simulink model "sim_sil_target_block"  (Simulink 8.1)
settings: Solver=FixedStepDiscrete  StartTime=0.0  StopTime=10.0  FixedStep=Auto  RelTol=1e-3  SampleTimeConstraint=STIndependent
undefined symbols (not defined in the file or in its folder): A10, A13, A14, B, B13, C6, D, D11, D4, K4, L3, PA10, PA11, PA12, PA13, PC6, PC7, R10
libraries: rappid_564xl_ec_toolbox x4, BAMLIB564xL x1
settings Model: Creator=evarshavskaya  LastModifiedBy=evarshavskaya  SimulationMode=software-in-the-loop (sil)
settings DataIOCC: ExternalInput=off  InitialState=off  SaveOutput=off  SignalLogging=off  SaveTime=off
settings OptimizationCC: InlineParams=on  OptimizeModelRefInitCode=on  LifeSpan=1
settings DebuggingCC: InheritedTsInSrcMsg=none  SingleTaskRateTransMsg=error  UnconnectedInputMsg=error  UnconnectedOutputMsg=error  UnconnectedLineMsg=error  UnknownTsInhSupMsg=error
settings HardwareCC: ProdIntDivRoundTo=Zero  ProdEndianess=LittleEndian  ProdHWDeviceType=Generic->Custom
settings ModelReferenceCC: ModelReferenceNumInstancesAllowed=Single
settings RTWCC: SystemTargetFile=ert.tlc  TemplateMakefile=ert_default_tmf  PostCodeGenCommand=rappid_analyzegencode(buildInfo)  Description=Embedded Coder  ProcessScript=ert_make_rtw_hook  PortableWordSizes=on  GenerateErtSFunction=on  CreateSILPILBlock=SIL  GenerateCodeInfo=on
settings CodeAppCC: IgnoreCustomStorageClasses=off  MaxIdLength=63  CustomSymbolStrType=$N$R$M  InternalIdentifier=Classic
settings ERTTargetCC: CodeReplacementLibrary=ANSI_C  MultiwordLength=2048  GenerateSampleERTMain=on  InlinedParameterPlacement=NonHierarchical  ERTCustomFileTemplate=example_file_process.tlc  ConvertIfToSwitch=off  SuppressUnreachableDefaultCases=off

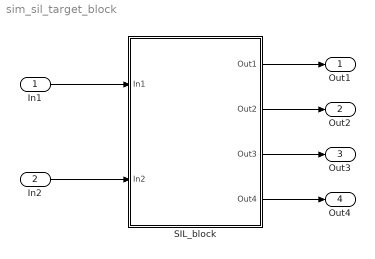
== system sim_sil_target_block ==
  In1 : Inport  OutDataTypeStr=uint16
  In2 : Inport  Port=2  OutDataTypeStr=single
  SIL_block : Subsystem
  Out1 : Outport
  Out2 : Outport  Port=2
  Out3 : Outport  Port=3
  Out4 : Outport  Port=4
  wires:
  In1/1 -> SIL_block/1(In1)
  In2/1 -> SIL_block/2(In2)
  SIL_block/2(Out2) -> Out2/1
  SIL_block/3(Out3) -> Out3/1
  SIL_block/4(Out4) -> Out4/1
  SIL_block/1(Out1) -> Out1/1

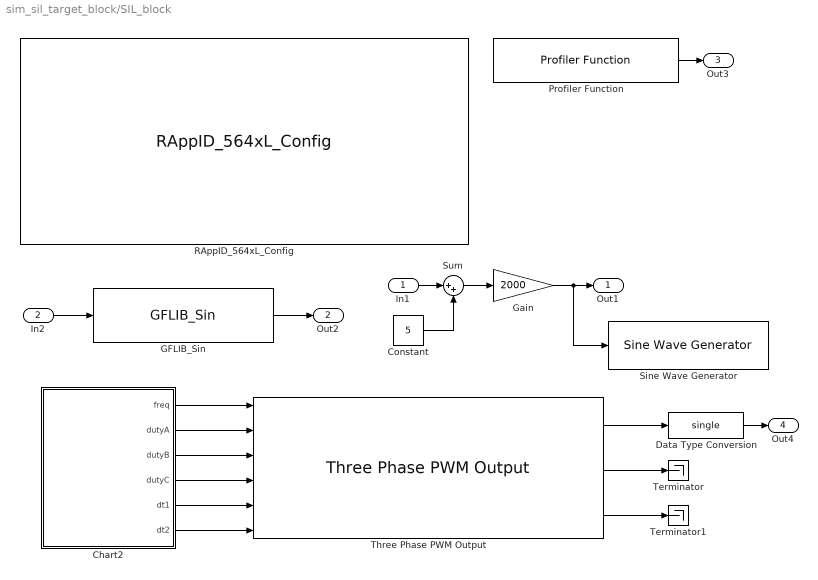
== system sim_sil_target_block/SIL_block ==
  In1 : Inport
  In2 : Inport  Port=2
  Chart2 : Stateflow chart  TreatAsAtomicUnit=on
  Constant : Constant  Value=5  OutDataTypeStr=uint16
  Data Type Conversion : DataTypeConversion  OutDataTypeStr=single
  GFLIB_Sin : BAMLIB564xL/General Functions/GFLIB_Sin
  Gain : Gain  Gain=2000  OutDataTypeStr=uint16
  "Profiler Function " : rappid_564xl_ec_toolbox/MPC564xL/Utility Blocks/Profiler Function   Priority=1  profile_indx=0
      settings: showOut=on
  RAppID_564xL_Config : rappid_564xl_ec_toolbox/MPC564xL/RAppID_564xL_Config  SystemClock=120  XTAL=40  MC_clock_60=12  MC_clock_80=16  MC_clock_120=10  SWG_clock_60=20  SWG_clock_80=13.334  SWG_clock_120=20  Compiler=CodeWarrior  MemTarget=RAM  Part=MPC5643L  Package=144 LQFP  global_int_priority=8  base_tick_priority=14  sys_task_supress=off  exception_handlers=off  stored_mdl_name=sim_sil_target_block  freemaster_interface=Oops  freemaster_rx_pin="LINFlex_0 Rx Pin 116 : \"PB[3]\""  freemaster_tx_pin="LINFlex_0 Tx Pin 114 : \"PB[2]\""  freemaster_interface_1=None  freemaster_enable=off  freemaster_rate=115200  freemaster_tx0_pin=18 : B[2] : 114 : A14  freemaster_rx0_pin=19 : B[3] : 116 : B13  freemaster_tx1_pin=57 : D[9] : 26 : L3  freemaster_rx1_pin=29 : B[13] : 60 : R10  freemaster_can_channel=1CH  freemater_can_speed=500K  freemaster_can_msgig=0x7AA  ccp_interface=None  ccp_enable=off  ccp_can_channel=CH1 (MB 0 - 1)  ccp_can_speed=500K  ccp_can_cro_id=256  ccp_can_dto_id=257  ccp_dev_id=RappID  ccp_dev_addr=0  ccp_odt=3  ccp_daq=3  pil_enable=on  pil_bam=on  comport=1  pil_rate=57600  bam_password_def=on  bam_password=0xFEEDFACECAFEBEEF  bam_sa_cs=off  bam_start_address=0x0  bam_code_size=0x7000  cons_dspi=on  cons_can=on  cons_adc=on  cons_pwm=on  cons_ctu=on  cons_swg=on  cons_eTimer=on  cons_fm=on
  Sine Wave Generator : rappid_564xl_ec_toolbox/MPC564xL/Motor Control Blocks/Sine Wave Generator  amplitude=2.097  frequency=2000  IOAMPL=14
  Sum : Sum  Inputs=|++  AccumDataTypeStr=int16
  Terminator : Terminator
  Terminator1 : Terminator
  Three Phase PWM Output : rappid_564xl_ec_toolbox/MPC564xL/Motor Control Blocks/Three Phase PWM Output  pwmModule=0  pwmMod=0  SubModule=0 1 2  subMod=0  InitFreq=1000  resolution=1 %  resValue=1  InitDutyA=75  InitDutyB=50  InitDutyC=25  DeadTime=100  dt=IPBus clock cycles  deadtime_mks=0  DebugSw=on  debug_mode=1  pin_A0="11  : PA11 : [ 120 ] : [ D11 ]"  pin_B0="10  : PA10 : [ 118 ] : [A13 ]"  pin_A1="39  : PC7  : [ 15 ] : [ K4 ]"  pin_B1="38  : PC6  : [ 142 ] : [ D4 ]"  pin_A2="12  : PA12 : [ 122 ] : [ A10 ]"  pin_B2="13  : PA13 : [ 136 ] : [ C6 ]"  pin_A3=None  pin_B3=None  pin1_A0=None  pin1_B0=None  pin1_A1=None  pin1_B1=None  pin1_A2=None  pin1_B2=None  pin1_A3=None  pin1_B3=None  pcrNum=0  polA0=off  polB0=off  polA1=off  polB1=off  polA2=off  polB2=off  polA3=off  polB3=off  octrl=0  outVal_A0=off  outVal_A1=off  outVal_A2=on  outVal_A3=on  outVal_B0=off  outVal_B1=off  outVal_B2=on  outVal_B3=on  outVal_C0=off  outVal_C1=off  outVal_C2=on  outVal_C3=on  outTrig=0
  Out1 : Outport
  Out2 : Outport  Port=2
  Out3 : Outport  Port=3
  Out4 : Outport  Port=4
  wires:
  Constant/1 -> Sum/2
  Sum/1 -> Gain/1
  Gain/1 -> Sine Wave Generator/1, Out1/1
  Chart2/1(freq) -> Three Phase PWM Output/1
  Chart2/2(dutyA) -> Three Phase PWM Output/2
  Chart2/3(dutyB) -> Three Phase PWM Output/3
  Chart2/4(dutyC) -> Three Phase PWM Output/4
  Chart2/5(dt1) -> Three Phase PWM Output/5
  Chart2/6(dt2) -> Three Phase PWM Output/6
  Three Phase PWM Output/1 -> Data Type Conversion/1
  Three Phase PWM Output/2 -> Terminator/1
  Three Phase PWM Output/3 -> Terminator1/1
  In1/1 -> Sum/1
  In2/1 -> GFLIB_Sin/1
  GFLIB_Sin/1 -> Out2/1
  "Profiler Function "/1 -> Out3/1
  Data Type Conversion/1 -> Out4/1

== stateflow chart SIL_block/Chart2 ==
  settings: executeAtInitialization=1
  state A
    en:
    freq =1000;
    dutyA=75;
    dutyB=50;
    dutyC=25;
    dt1=200;
    dt2=200;
    du:
    cntr=cntr+1;
  state A1
    en:
    freq =1000;
    dutyA=25;
    dutyB=75;
    dutyC=50;
    dt1=200;
    dt2=200;
    du:
    cntr=cntr+1;
  state A2
    en:
    freq =1000;
    dutyA=50;
    dutyB=25;
    dutyC=75;
    dt1=200;
    dt2=200;
    du:
    cntr=cntr+1;
    ex:
    cntr = 0;
  (default) -> A : {cntr=0;}
  A2 -> A : [cntr > 30]
  A -> A1 : [cntr > 10]
  A1 -> A2 : [cntr > 20]
  data: cntr local uint32 =0; freq output uint32; dutyA output uint32; dutyB output uint32; dutyC output uint32; dt1 output uint32; dt2 output uint32
